simulink model "walkingRobot_Forward2"  (R2018a)
settings: Solver=FixedStepAuto  StartTime=0.0  StopTime=5  FixedStep=.01  MinStep=.005  EnableMultiTasking=on
model workspace (MAT data in the model file):
  MCOS : class17 (value not decoded)
values from neighbouring files (symbols this model uses):
  Am = repmat(Am,1,6/length(Am))    [CostFCN.m]    (also in learn_rcp_batch.m = 1; optimizeRobotMotion_openLoop.m; pFinal_runSim.m; runSim_testParams.m = ones(1,6))
  ankle_servo_kd = 8    [robotParameters.m]
  ankle_servo_ki = 4    [robotParameters.m]
  ankle_servo_kp = 20    [robotParameters.m]
  contact_damping = 2200    [robotParameters.m]
  contact_point_radius = .005    (= 0.005)    [robotParameters.m]
  contact_stiffness = 300    [robotParameters.m]
  deriv_filter_coeff = 100    [robotParameters.m]
  height_plane = 0.1    [robotParameters.m]
  hip_servo_kd = 20    [robotParameters.m]
  hip_servo_ki = 10    [robotParameters.m]
  hip_servo_kp = 60    [robotParameters.m]
  init_pos = Am'.*init_pos    [CostFCN.m]    (also in optimizeRobotMotion_openLoop.m; pFinal_runSim.m; simWalker_constraint.m)
  init_vel = Am'.*init_vel    [CostFCN.m]    (also in optimizeRobotMotion_openLoop.m; pFinal_runSim.m; simWalker_constraint.m)
  joint_damping = 0    [robotParameters.m]
  joint_stiffness = 0    [robotParameters.m]
  knee_servo_kd = 10    [robotParameters.m]
  knee_servo_ki = 5    [robotParameters.m]
  knee_servo_kp = 60    [robotParameters.m]
  max_torque = 20    [robotParameters.m]
  motion_time_constant = 0.01    [robotParameters.m]
  motor_constant = 0.02    [robotParameters.m]
  motor_inertia = 0    [robotParameters.m]
  mu_k = 0.5    [robotParameters.m]
  mu_s = .6    (= 0.6)    [robotParameters.m]
  mu_vth = 0.1    [robotParameters.m]
  plane_x = 3    [robotParameters.m]
  plane_y = .3    (= 0.3)    [robotParameters.m]
  tau = params(1,2)    [CostFCN.m]    (also in Test_params.m = tau_nom; Trajectory.m = (2*pi)/omega; learn_rcp_batch.m = 1.13; optimizeRobotMotion_openLoop.m = pFinal(1,2))
  Traj = Am.*init_pos'*pi/180    [CostFCN.m]    (also in Test_params.m = init_pos'*pi/180; learn_rcp_batch.m = zeros(1,6); optimizeRobotMotion_openLoop.m; pFinal_runSim.m)
  upper_leg_length = 38    [robotParameters.m]
  V_treadmill = 0.3 + (1.7/5)*(k-1)    [optimizeRobotMotion_openLoop.m]    (also in pFinal_runSim.m = .3+(j-1)*1.7/5; runSim_testParams.m = 1)
  W = [DMP(1).w DMP(2).w DMP(3).w DMP(4).w DMP(5).w DMP(6).w]    [learn_rcp_batch.m]
  Ym = Ym.*Am    [CostFCN.m]    (also in learn_rcp_batch.m = [DMP(1).ym DMP(2).ym DMP(3).ym DMP(4).ym DMP(5).ym DMP(6).ym; optimizeRobotMotion_openLoop.m; pFinal_runSim.m; simWalker_constraint.m)
undefined symbols (not defined in the file or in its folder): Extr_Data_LinkHoles, X, Y, YBT_Par, Z
libraries: nesl_utility x155, sm_lib x136, Contact_Forces_Lib x34, simulink x28, fl_lib x14, Parts_Lib x10, elec_lib x6, walkingRobotUtils x5, simulink_extras x2, Multibody_Multiphysics_Lib x2
(part 10 of 10)

== system walkingRobot_Forward2/Robot/Robot Leg R/Box to Belt In Force/Sphere to Plane Force Enabled nz4/Forces/Ff/SlipVel ==
  wx : Inport
  wy : Inport  Port=2
  vx : Inport  Port=3
  vy : Inport  Port=4
  Fx1 : Constant  Value=sphere_rad
  Math Function : Math  Operator=square  SaturateOnIntegerOverflow=on
  Math Function1 : Math  Operator=square  SaturateOnIntegerOverflow=on
  Product3 : Product
  Product4 : Product
  Sqrt : Sqrt  SaturateOnIntegerOverflow=on
  Sum1 : Sum  Inputs=|++
  Sum2 : Sum  Inputs=|-+
  Sum3 : Sum  Inputs=|++
  Trigonometric Function : Trigonometry  Operator=atan2
  vabs : Outport
  alpha : Outport  Port=2
  wires:
  wx/1 -> Product3/1
  Product3/1 -> Sum1/1
  wy/1 -> Product4/2
  vx/1 -> Sum2/2
  Fx1/1 -> Product3/2, Product4/1
  vy/1 -> Sum1/2
  Product4/1 -> Sum2/1
  Trigonometric Function/1 -> alpha/1
  Sqrt/1 -> vabs/1
  Sum3/1 -> Sqrt/1
  Math Function/1 -> Sum3/1
  Math Function1/1 -> Sum3/2
  Sum1/1 -> Trigonometric Function/1, Math Function/1  "slipy"
  Sum2/1 -> Trigonometric Function/2, Math Function1/1  "slipx"

== system walkingRobot_Forward2/Robot/Robot Leg R/Box to Belt In Force/Sphere to Plane Force Enabled nz5/Forces/Ff/SlipVel ==
  wx : Inport
  wy : Inport  Port=2
  vx : Inport  Port=3
  vy : Inport  Port=4
  Fx1 : Constant  Value=sphere_rad
  Math Function : Math  Operator=square  SaturateOnIntegerOverflow=on
  Math Function1 : Math  Operator=square  SaturateOnIntegerOverflow=on
  Product3 : Product
  Product4 : Product
  Sqrt : Sqrt  SaturateOnIntegerOverflow=on
  Sum1 : Sum  Inputs=|++
  Sum2 : Sum  Inputs=|-+
  Sum3 : Sum  Inputs=|++
  Trigonometric Function : Trigonometry  Operator=atan2
  vabs : Outport
  alpha : Outport  Port=2
  wires:
  Sum2/1 -> Math Function1/1, Trigonometric Function/2  "slipx"
  Sum1/1 -> Math Function/1, Trigonometric Function/1  "slipy"
  Math Function1/1 -> Sum3/2
  Math Function/1 -> Sum3/1
  Sum3/1 -> Sqrt/1
  Sqrt/1 -> vabs/1
  Trigonometric Function/1 -> alpha/1
  Product4/1 -> Sum2/1
  vy/1 -> Sum1/2
  Fx1/1 -> Product4/1, Product3/2
  vx/1 -> Sum2/2
  wy/1 -> Product4/2
  Product3/1 -> Sum1/1
  wx/1 -> Product3/1

== matlab function walkingRobot_Forward2/Robot/Robot Leg R/MATLAB Function ==
  data: f0 input; f1 input; y output
function y = fcn(f0, f1)
y = (f0==0 && f1>0);

== matlab function walkingRobot_Forward2/Robot/DMP Generation/Forcing_Term2 ==
  data: f output; PSI input; W input; Amp input
function f = fcn(PSI,W,Amp)

f = zeros(1,6);

for i=1:6
%     amp = Amp(i);
    w   = W(:,i);
    psi = PSI(:,i);
    A = Amp(i);
    
    f(i)            = sum(w.*psi)/sum(psi+1.e-10) * A;
    
end
end

== matlab function walkingRobot_Forward2/Robot/DMP Generation/Gaussian_fun2 ==
  data: PSI output; Phi input
function PSI = fcn(Phi)

n_rfs  = 100;    % number of kernel functions

% the time constants for chosen for critical damping

c       = 2*pi*(1/n_rfs:1/n_rfs:1)';
D       = ones(n_rfs,1)*.1*n_rfs^2;

PSI = zeros(n_rfs,6);

for i=1:6
    
    p = Phi;
    
    PSI(:,i) = exp(D.*(cos(p-c)-1));
    
end

== matlab function walkingRobot_Forward2/Robot/DMP Generation/Initial States ==
  data: tau input; pos_i output; init_pos input; init_vel input; z_i output
function [pos_i, z_i] = fcn(tau,init_pos,init_vel)

pos_i = zeros(6,1);
z_i   = zeros(6,1);
for i=1:6

    pos_i(i,1)   = init_pos(i,1);
    vel_i   = init_vel(i,1);
    z_i(i,1)     = vel_i*tau;
        
end
    
end

== matlab function walkingRobot_Forward2/Robot/DMP Generation/DMP+Initiation4 ==
  data: t input; init_pos input; DMP_rev output; Y input
function DMP_rev = fcn(t, init_pos, Y)

yy = 0;

for j = 1:6
    
    %% Knee Trajectories saturation
    if j==2 || j==5
        if Y(j)<0
            Y(j) = 0;
        end
    end
    
    %% Smoothening of the Hip Trajectories Notches
%     if t>156*dt && t<174*dt
%         
%         if j==1 || j==4
%             if t == 156*dt
%                 yy = Y(j);
%             end
%             
%             Y(j)=yy+(Y(j)-yy)*(t/dt-156)'/17;
%         end
%     end
    
    %% Set up the initial trajectory bridging the double-stance phase to the onset of the DMP Trajectory
%     if t<=.01
%         if j==1
%             Y(j) = 0;
%         elseif j==2
%             Y(j) = 0;
%         elseif j==4
%             Y(j) = 0;
%         elseif  j==3 || j==6
%             Y(j) = 0;
%         elseif j==5
%             Y(j) = 0;
%         end
%         
%     %%%    
% %     elseif t<=.59
% %         if j==1
% %             Y(j) = -22.09*t/.59;
% %         elseif j==2
% %             Y(j) = 5.86*t/.59;
% %         elseif j==4     % right hip in orange
% %             Y(j) = -4.7*t/.59;
% %         elseif  j==3 || j==6    % 6: right ankle in yellow
% %             Y(j) = 0;
% %         elseif j==5     % right knee in blue
% %             Y(j) = -(6/.29^2)*(t-.29).^2+3;
% %             if Y(j)<0
% %                 Y(j)=0;
% %             end
% %             
% % 
% %         end
%        %%%% 
% %     elseif t>.45 && t<=.475
% %         Y(4)=4.7-(t-.45)/.025*.75;
%     %%%%    
%     elseif t<=.67
%         if j==1
%             Y(j) = +23/(.39)^2*(t-.39).^2-23;
%         elseif j==4
%             Y(j) = 5*t/.65;
%         elseif  j==3   % 6: right ankle in yellow
%             Y(j) = -0*t/.65;
%         elseif  j==6   % 6: right ankle in yellow
%             Y(j) = 0;
%         elseif j==2
%             Y(j)= 14*t/.6;
%             
%         elseif j==5     % right knee in blue
%             Y(j) = -(10/.29^2)*(t-.29).^2+10;
%             if Y(j)<0
%                 Y(j)=0;
%             end
%             
% 
%         end
%     %%%%%    
%     end
    
    %% The final revised DMP
    DMP_rev = Y(end:-1:1);
end
